simulink model "Requirements_Table"  (R2022a)
settings: Solver=FixedStepAuto  StartTime=0.0  StopTime=10.0  FixedStep=1e-3  RelTol=1e-3  EnableMultiTasking=on
settings Model: ExtModeTrigDuration=5  Creator=tygre  LastModifiedBy=tygre
settings OptimizationCC: EnhancedBackFolding=on  PassReuseOutputArgsAs=Individual arguments  ZeroExternalMemoryAtStartup=off  ZeroInternalMemoryAtStartup=off  MaxStackSize=64  OptimizeBlockOrder=speed  DifferentSizesBufferReuse=on  OptimizationCustomize=off  EfficientTunableParamExpr=on
settings DebuggingCC: ParameterTunabilityLossMsg=error
settings HardwareCC: ProdBitPerPointer=32  ProdBitPerSizeT=32  ProdBitPerPtrDiffT=32  ProdLargestAtomicInteger=Long  ProdLargestAtomicFloat=Double  ProdWordSize=32  ProdHWDeviceType=ARM Compatible->ARM Cortex
settings SFSimCC: MATLABDynamicMemAlloc=off
settings RTWCC: SystemTargetFile=ert.tlc  HardwareBoard=NXP FRDM-K64F  TLCOptions="-aInlineSetEventsForThisBaseRateFcn=TLC_FALSE -aSuppressMultiTaskScheduler=TLC_FALSE  -aRateBasedStepFcn=0"  TemplateMakefile=ert_default_tmf  Toolchain=GNU Tools for ARM Embedded Processors
settings CodeAppCC: ForceParamTrailComments=on  IgnoreCustomStorageClasses=off  OperatorAnnotations=on  SimulinkDataObjDesc=on  SFDataObjDesc=on  InsertBlockDesc=on
settings ERTTargetCC: ExtModeTransport=4  ExtModeMexFile=sendToCommService

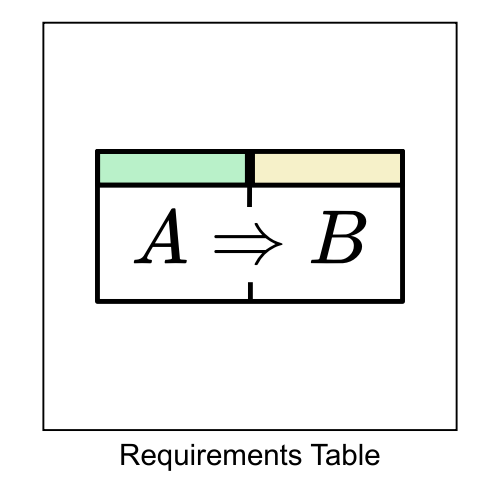
[thumbnail: Simulink's stored preview of the top-level diagram]
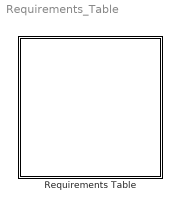
== system Requirements_Table ==
  Requirements Table : Requirements Table  TreatAsAtomicUnit=on

== stateflow chart Requirements_Table/Requirements Table ==
  (default) -> (junction 1073743818)
  (junction 1073743818) -> (junction 1073743819) : {
      | % SF_REQ_REV_07
      | }
  (junction 1073743819) -> (junction 1073743821) : {
      | % HEADER_ASSIGNMENTS
      |
      | }
  (junction 1073743821) -> (junction 1073743823) : {
      | % START_A_4
      | }
  (junction 1073743823) -> (junction 1073743825) : {
      | }
  (junction 1073743825) -> (junction 1073743827)
  (junction 1073743827) -> (junction 1073743829) : {
      | }
  (junction 1073743829) -> (junction 1073743831) : {
      | % END_A_4
      | }
  (junction 1073743831) -> (junction 1073743833) : {
      | % START_R_1
      | }
  (junction 1073743833) -> (junction 1073743835) : {
      | }
  (junction 1073743835) -> (junction 1073743837)
  (junction 1073743837) -> (junction 1073743839) [order 1] : [(PACE_CHARGE_CTRL==false) && (PACE_GND_CTRL==true) && (VENT_GND_CTRL==false) && (VENT_PACE_CTRL==true)]
  (junction 1073743837) -> (junction 1073743845) [order 2]
  (junction 1073743839) -> (junction 1073743841) : {
      | reqtable_postcondition((PACE_CHARGE_CTRL==true) && (PACE_GND_CTRL==true) && (VENT_GND_CTRL==true) && (VENT_PACE_CTRL==false), 'R:1');
      |
      |
      | }
  (junction 1073743841) -> (junction 1073743843) : {
      | }
  (junction 1073743843) -> (junction 1073743845)
  (junction 1073743845) -> (junction 1073743847)
  (junction 1073743847) -> (junction 1073743849) : {
      | % END_R_1
      | }
  (junction 1073743849) -> (junction 1073744013) : {
      | % START_R_43
      | }
  (junction 1073744013) -> (junction 1073744015) : {
      | }
  (junction 1073744015) -> (junction 1073744017)
  (junction 1073744017) -> (junction 1073744019) [order 1] : [(PACE_GND_CTRL==true) && (Mode==VVI) && (VENT_CMP_DETECT==true)]
  (junction 1073744017) -> (junction 1073744025) [order 2]
  (junction 1073744019) -> (junction 1073744021) : {
      | reqtable_postcondition((PACE_CHARGE_CTRL==true) && (PACE_GND_CTRL==true) && (VENT_GND_CTRL==true) && (VENT_PACE_CTRL==false), 'R:2');
      |
      |
      | }
  (junction 1073744021) -> (junction 1073744023) : {
      | }
  (junction 1073744023) -> (junction 1073744025)
  (junction 1073744025) -> (junction 1073744027)
  (junction 1073744027) -> (junction 1073744029) : {
      | % END_R_43
      | }
  (junction 1073744029) -> (junction 1073743851) : {
      | % START_R_13
      | }
  (junction 1073743851) -> (junction 1073743853) : {
      | }
  (junction 1073743853) -> (junction 1073743855)
  (junction 1073743855) -> (junction 1073743857) [order 1] : [(PACE_CHARGE_CTRL==true) && (PACE_GND_CTRL==true) && (VENT_GND_CTRL==true) && (VENT_PACE_CTRL==false) && (Mode~=VVI)]
  (junction 1073743855) -> (junction 1073743863) [order 2]
  (junction 1073743857) -> (junction 1073743859) : {
      | reqtable_postcondition((PACE_CHARGE_CTRL==false) && (PACE_GND_CTRL==true) && (VENT_GND_CTRL==false) && (VENT_PACE_CTRL==true), 'R:3');
      |
      |
      | }
  (junction 1073743859) -> (junction 1073743861) : {
      | }
  (junction 1073743861) -> (junction 1073743863)
  (junction 1073743863) -> (junction 1073743865)
  (junction 1073743865) -> (junction 1073743867) : {
      | % END_R_13
      | }
  (junction 1073743867) -> (junction 1073743869) : {
      | % START_R_16
      | }
  (junction 1073743869) -> (junction 1073743871) : {
      | }
  (junction 1073743871) -> (junction 1073743873)
  (junction 1073743873) -> (junction 1073743875) [order 1] : [(PACE_CHARGE_CTRL==false) && (PACE_GND_CTRL==true) && (ATR_GND_CTRL==false) && (ATR_PACE_CTRL==true)]
  (junction 1073743873) -> (junction 1073743881) [order 2]
  (junction 1073743875) -> (junction 1073743877) : {
      | reqtable_postcondition((PACE_CHARGE_CTRL==true) && (PACE_GND_CTRL==true) && (ATR_GND_CTRL==true) && (ATR_PACE_CTRL==false), 'R:4');
      |
      |
      | }
  (junction 1073743877) -> (junction 1073743879) : {
      | }
  (junction 1073743879) -> (junction 1073743881)
  (junction 1073743881) -> (junction 1073743883)
  (junction 1073743883) -> (junction 1073743885) : {
      | % END_R_16
      | }
  (junction 1073743885) -> (junction 1073744034) : {
      | % START_R_46
      | }
  (junction 1073744034) -> (junction 1073744036) : {
      | }
  (junction 1073744036) -> (junction 1073744038)
  (junction 1073744038) -> (junction 1073744040) [order 1] : [(PACE_GND_CTRL==true) && (Mode==AAI) && (ATR_CMP_DETECT==true)]
  (junction 1073744038) -> (junction 1073744046) [order 2]
  (junction 1073744040) -> (junction 1073744042) : {
      | reqtable_postcondition((PACE_CHARGE_CTRL==true) && (PACE_GND_CTRL==true) && (ATR_GND_CTRL==true) && (ATR_PACE_CTRL==false), 'R:5');
      |
      |
      | }
  (junction 1073744042) -> (junction 1073744044) : {
      | }
  (junction 1073744044) -> (junction 1073744046)
  (junction 1073744046) -> (junction 1073744048)
  (junction 1073744048) -> (junction 1073744050) : {
      | % END_R_46
      | }
  (junction 1073744050) -> (junction 1073743887) : {
      | % START_R_19
      | }
  (junction 1073743887) -> (junction 1073743889) : {
      | }
  (junction 1073743889) -> (junction 1073743891)
  (junction 1073743891) -> (junction 1073743893) [order 1] : [(PACE_CHARGE_CTRL==true) && (PACE_GND_CTRL==true) && (ATR_GND_CTRL==true) && (ATR_PACE_CTRL==false) && (Mode~=AAI)]
  (junction 1073743891) -> (junction 1073743899) [order 2]
  (junction 1073743893) -> (junction 1073743895) : {
      | reqtable_postcondition((PACE_CHARGE_CTRL==false) && (PACE_GND_CTRL==true) && (ATR_GND_CTRL==false) && (ATR_PACE_CTRL==true), 'R:6');
      |
      |
      | }
  (junction 1073743895) -> (junction 1073743897) : {
      | }
  (junction 1073743897) -> (junction 1073743899)
  (junction 1073743899) -> (junction 1073743901)
  (junction 1073743901) -> (junction 1073743903) : {
      | % END_R_19
      | }
  (junction 1073743903) -> (junction 1073743905) : {
      | % START_R_22
      | }
  (junction 1073743905) -> (junction 1073743907) : {
      | }
  (junction 1073743907) -> (junction 1073743909)
  (junction 1073743909) -> (junction 1073743911) [order 1] : [(PACE_CHARGE_CTRL==true) && (PACE_GND_CTRL==true) && (VENT_GND_CTRL==true) && (VENT_PACE_CTRL==false) && (Mode==VVI)]
  (junction 1073743909) -> (junction 1073743917) [order 2]
  (junction 1073743911) -> (junction 1073743913) : {
      | reqtable_postcondition((FRONTEND_CTRL==true), 'R:7');
      |
      |
      | }
  (junction 1073743913) -> (junction 1073743915) : {
      | }
  (junction 1073743915) -> (junction 1073743917)
  (junction 1073743917) -> (junction 1073743919)
  (junction 1073743919) -> (junction 1073743921) : {
      | % END_R_22
      | }
  (junction 1073743921) -> (junction 1073743923) : {
      | % START_R_34
      | }
  (junction 1073743923) -> (junction 1073743925) : {
      | }
  (junction 1073743925) -> (junction 1073743927)
  (junction 1073743927) -> (junction 1073743929) [order 1] : [(PACE_CHARGE_CTRL==true) && (PACE_GND_CTRL==true) && (ATR_GND_CTRL==true) && (ATR_PACE_CTRL==false) && (Mode==AAI)]
  (junction 1073743927) -> (junction 1073743935) [order 2]
  (junction 1073743929) -> (junction 1073743931) : {
      | reqtable_postcondition((FRONTEND_CTRL==true), 'R:8');
      |
      |
      | }
  (junction 1073743931) -> (junction 1073743933) : {
      | }
  (junction 1073743933) -> (junction 1073743935)
  (junction 1073743935) -> (junction 1073743937)
  (junction 1073743937) -> (junction 1073743969) : {
      | % END_R_34
      | }
